simulink model "sys_model"  (R2015a)
settings: configuration reference "config_cosim" (kept outside this file)
InitFcn:
  | h  = findall(0, 'tag','Display');
  | close(h)
  | load TestVel
StartFcn:
  | Display
StopFcn:
  | h  = findall(0, 'tag','Display');
  | %close(h)
undefined symbols (not defined in the file): Vmsl, Vtgt
(part 2 of 2)

== stateflow chart sys_model/CC_module/Subsystem/DisplayControl ==
  settings: executeAtInitialization=1
  state Init
    entry:
    TargetData= TargetDataLD;
    AsnData = zeros(8,2)
    StateData = zeros(8,3);
    StateInf = 0;
    avl_asn_msl = ones(8,1);
    avl_FS_tgt = ones(8,1);
    avl_pwr_tgt = ones(8,1);
  state On
    state TargetPower [parallel]
      % 根据选择的目标更新加电和断电信息
      settings: executionOrder=4
      TargetPower -> (junction 337)
      (junction 337) -> (junction 441) [order 1] : [Actions.TgtAsn]
      (junction 337) -> (junction 339) [order 2]
      (junction 441) -> (junction 443) : {avl_pwr_tgt(Inds.TgtAsnInd) = 1;}
      (junction 443) -> (junction 339)
      (junction 339) -> (junction 687)
      (junction 687) -> (junction 685) [order 1] : [Actions.TgtAsnCcl]
      (junction 687) -> (junction 684) [order 2]
      (junction 685) -> (junction 691) : {avl_pwr_tgt(Inds.TgtAsnInd) = 0;}
      (junction 691) -> (junction 684)
    state DataProcess [parallel]
      en:
      %info2FSC.Para_FS(1:8) = 0;
      Para_FS0.pos_tgt = [0;0;0];
      Para_FS0.vel_tgt = [0;0;0];
      info2FSC.Para_FS(1:8) = Para_FS0;
      info2FSC.ins_pwr_on =  false(8,1);
      info2FSC.ins_pwr_of = [false;false;false;false;false;false;false;false];
      info2FSC.ins_FS = [false;false;false;false;false;false;false;false];
      settings: executionOrder=6
      state PwrOff [parallel]
        settings: executionOrder=3
        (default) -> (junction 889)
        On.DataProcess.PwrOff -> (junction 889)
        (junction 889) -> (junction 880) [order 1] : [Actions.PwrOff]
        (junction 889) -> (junction 1219) [order 2]
        (junction 880) -> (junction 1217) : {info2FSC.ins_pwr_on = [false;false;false;false;false;false;false;false];
            | info2FSC.ins_pwr_of =Inds.PwrInd;
            | info2FSC.ins_FS = [false;false;false;false;false;false;false;false];}
        (junction 1217) -> (junction 1219)
        (junction 1219) -> (junction 1382)
      state PwrOn [parallel]
        settings: executionOrder=1
        (default) -> (junction 863)
        (junction 863) -> (junction 852) [order 1] : [Actions.PwrOn]
        On.DataProcess.PwrOn -> (junction 863)
        (junction 863) -> (junction 1212) [order 2]
        (junction 852) -> (junction 1214) : {info2FSC.ins_pwr_on = Inds.PwrInd;
            | info2FSC.ins_pwr_of = [false;false;false;false;false;false;false;false];
            | info2FSC.ins_FS = [false;false;false;false;false;false;false;false];}
        (junction 1214) -> (junction 1212)
        (junction 1212) -> (junction 1380)
      state FS [parallel]
        settings: executionOrder=2
        (default) -> (junction 914)
        On.DataProcess.FS -> (junction 914)
        (junction 914) -> (junction 905) [order 1] : [Actions.FS]
        (junction 914) -> (junction 1222) [order 2]
        (junction 905) -> (junction 902) : {info2FSC.ins_pwr_on = [false;false;false;false;false;false;false;false];
            | info2FSC.ins_pwr_of = [false;false;false;false;false;false;false;false];
            | info2FSC.ins_FS = [false;false;false;false;false;false;false;false];}
        (junction 913) -> (junction 922) [order 1] : [Inds.TgtFsInd(i,1)]
        (junction 1221) -> (junction 913) [order 1] : [i  < 9]
        (junction 902) -> (junction 1221) : {i = 1;}
        (junction 913) -> (junction 907) [order 2]
        (junction 922) -> (junction 1201) : {ddInd1 = AsnData(i,1);
            | info2FSC.ins_FS(ddInd1) = true;}
        (junction 1201) -> (junction 907)
        (junction 907) -> (junction 919)
        (junction 1221) -> (junction 1222) [order 2]
        (junction 916) -> (junction 1221) : {i = i + 1;}
        (junction 1222) -> (junction 1384)
        (junction 919) -> (junction 918) [order 1] : [Inds.TgtFsInd(i,2)]
        (junction 918) -> (junction 1203) : {ddInd1 = AsnData(i,2);
            | info2FSC.ins_FS(ddInd1) = true;}
        (junction 919) -> (junction 916) [order 2]
        (junction 1203) -> (junction 916)
      state DataUpdateWithFSCInfo [parallel]
        settings: executionOrder=4
        state Enter
        state Sub
          (default) -> (junction 981)
          (junction 981) -> (junction 980) : {avl_asn_msl =double(avl_asn_msl&info_FSC.avl_msl);
              | m = 0;
              | n = 0;
              | j = 1;}
          (junction 979) -> (junction 968) [order 1] : % 导弹出现故障
              | [~info_FSC.avl_msl(j)]
          (junction 980) -> (junction 979) [order 1] : [j  < 9]
          (junction 979) -> (junction 972) [order 2]
          (junction 968) -> (junction 994) : {StateData(j,1:3) =2;}
          (junction 972) -> (junction 984) [order 1] : %虽然有加电命令，但是加电状态为未加电
              | [info2FSC.ins_pwr_on(j)==1 && info_FSC.stt_pwr_msl(j) ==0]
          (junction 977) -> (junction 980) : {j = j + 1;}
          (junction 980) -> (junction 999) [order 2]
          (junction 972) -> (junction 973) [order 2]
          (junction 984) -> (junction 988) : {StateData(j,2) = 0;
              | m = m+1;}
          (junction 973) -> (junction 966) [order 1] : %虽然有发射命令，但是离架计时为0，说明没有发生
              | [info2FSC.ins_FS(j)==1 && info_FSC.count_sprt_msl(j)<=0]
          (junction 973) -> (junction 977) [order 2]
          (junction 966) -> (junction 991) : {StateData(j,3) = 0;
              | n = n+1;}
          (junction 991) -> (junction 977)
          (junction 988) -> (junction 991)
          (junction 994) -> (junction 988)
          (junction 999) -> (junction 1001) [order 1] : [sum(info2FSC.ins_pwr_on)>0&&StateInf~= 712]
          (junction 1001) -> (junction 1350) [order 1] : % 说明本次没有加电成功的DD
              | [m == sum(info2FSC.ins_pwr_on)]
          (junction 999) -> (junction 1005) [order 2]
          (junction 1001) -> (junction 1003) [order 2] : {StateInf = 710;}
          (junction 1350) -> (junction 1352) : {StateInf = 712;}
          (junction 1003) -> (junction 1005)
          (junction 1352) -> (junction 1003)
          (junction 1005) -> (junction 1368)
          (junction 1368) -> (junction 1369) [order 1] : [sum(info2FSC.ins_pwr_of)>0]
          (junction 1368) -> (junction 1370) [order 2]
          (junction 1369) -> (junction 1371) : {StateInf = 810;}
          (junction 1371) -> (junction 1370)
          (junction 1370) -> (junction 1009)
          (junction 1009) -> (junction 1491) [order 1] : [sum(info2FSC.ins_FS)>0]
          (junction 1491) -> (junction 1011) [order 1] : [n == sum(info2FSC.ins_FS)] % 说明本次没有发射成功的DD
          (junction 1009) -> (junction 1008) [order 2]
          (junction 1491) -> (junction 1493) [order 2] : {StateInf = 112;}
          (junction 1011) -> (junction 1012) : {StateInf = 110;}
          (junction 1493) -> (junction 1008)
          (junction 1012) -> (junction 1493)
          (junction 1008) -> (junction 1021) : {StateData0.StateData = StateData;
              | StateData0.StateInf = StateInf;
              | avl_FS_tgt = avl_FS_tgt0;}
        state Waiting
          en:StateInf = 0;
        (default) -> On.DataProcess.DataUpdateWithFSCInfo.Enter
        On.DataProcess.DataUpdateWithFSCInfo.Enter -> On.DataProcess.DataUpdateWithFSCInfo.Waiting : [Actions.PwrOn||Actions.PwrOff||Actions.FS]
        On.DataProcess.DataUpdateWithFSCInfo.Waiting -> Sub : [after(1,tick)]
        Sub -> DataUpdateWithFSCInfo
    state TargetDataProcess [parallel]
      settings: executionOrder=1
      state Time
      (default) -> Time : { TargetData = TargetDataLD;}
      Time -> TargetDataProcess : [after(0.001,sec)]
    state DataUpdate [parallel]
      % 根据状态更新状态信息以及表格中要显示的数据
      en:StateData = zeros(8,3);
      settings: executionOrder=2
      state Assign [parallel]
        settings: executionOrder=1
        Assign -> (junction 412)
        (junction 412) -> (junction 416) [order 1] : [Actions.TgtAsn]
        (junction 412) -> (junction 415) [order 2]
        (junction 416) -> (junction 410) : {AsnData(Inds.TgtAsnInd,1) = Inds.MslInd(1);
            |  AsnData(Inds.TgtAsnInd,2) = Inds.MslInd(2);}
        (junction 410) -> (junction 447) [order 1] : [Inds.MslInd(1)]
        (junction 410) -> (junction 815) [order 2]
        (junction 447) -> (junction 814) : {StateData(Inds.MslInd(1),2)= 1;}
        (junction 814) -> (junction 815)
        (junction 815) -> (junction 449)
        (junction 449) -> (junction 452) [order 1] : [Inds.MslInd(2)]
        (junction 449) -> (junction 454) [order 2]
        (junction 452) -> (junction 818) : {StateData(Inds.MslInd(2),2) = 1;}
        (junction 454) -> (junction 415)
        (junction 818) -> (junction 454)
        (junction 415) -> (junction 662)
        (junction 662) -> (junction 664) [order 1] : [Actions.TgtAsnCcl]
        (junction 662) -> (junction 665) [order 2]
        (junction 664) -> (junction 1518) : {AsnData(Inds.TgtAsnInd,1) = 0;
            |  AsnData(Inds.TgtAsnInd,2) = 0;}
        (junction 1518) -> (junction 1512) [order 1] : [Inds.MslInd(1)]
        (junction 1518) -> (junction 1510) [order 2]
        (junction 1512) -> (junction 1520) : {StateData(Inds.MslInd(1),2) = 0;}
        (junction 1520) -> (junction 1510)
        (junction 1510) -> (junction 1504)
        (junction 1504) -> (junction 1503) [order 1] : [Inds.MslInd(2)]
        (junction 1504) -> (junction 1517) [order 2]
        (junction 1503) -> (junction 1516) : {StateData(Inds.MslInd(2),2) = 0;}
        (junction 1517) -> (junction 665)
        (junction 1516) -> (junction 1517)
        (junction 665) -> (junction 1360) : {StateData0.StateData = StateData;
            | StateData0.StateInf = 0;}
      state PwrOn [parallel]
        settings: executionOrder=2
        state PowerOn
          (default) -> (junction 532) : {i = 1;}
          (junction 544) -> (junction 543) [order 1] : [PwrInd(i)]
          (junction 532) -> (junction 544) [order 1] : [i  < 9]
          (junction 544) -> (junction 545) [order 2]
          (junction 543) -> (junction 542) : {StateData(i,1) = 1;}
          (junction 545) -> (junction 532) : {i = i + 1;}
          (junction 542) -> (junction 545)
          (junction 532) -> (junction 1229) [order 2]
        state Enter
        state Waiting
          entry:
          PwrInd = Inds.PwrInd;
        (default) -> On.DataUpdate.PwrOn.Enter
        On.DataUpdate.PwrOn.Enter -> On.DataUpdate.PwrOn.Waiting : [Actions.PwrOn]
        On.DataUpdate.PwrOn.Waiting -> PowerOn : [after(1,tick)]
        PowerOn -> On.DataUpdate.PwrOn
      state FS [parallel]
        settings: executionOrder=4
        state Enter3
        state Waiting3
          entry:
          TgtFsInd = Inds.TgtFsInd;
        state fs
          (junction 611) -> (junction 604) [order 1] : [i  < 9]
          (junction 604) -> (junction 607)
          (default) -> (junction 611) : {i = 1;}
          (junction 607) -> (junction 608) [order 1] : [TgtFsInd(i,1)>0]
          (junction 607) -> (junction 609) [order 2]
          (junction 608) -> (junction 610) : {ddInd = AsnData(i,1);
              | StateData(ddInd,3) = 1;}
          (junction 610) -> (junction 609)
          (junction 609) -> (junction 612)
          (junction 617) -> (junction 611) : {i = i + 1;}
          (junction 611) -> (junction 616) [order 2]
          (junction 612) -> (junction 613) [order 1] : [TgtFsInd(i,2)>0]
          (junction 612) -> (junction 614) [order 2]
          (junction 613) -> (junction 615) : {ddInd = AsnData(i,2);
              | StateData(ddInd,3) = 1;}
          (junction 615) -> (junction 614)
          (junction 614) -> (junction 617)
        (default) -> Enter3
        Enter3 -> Waiting3 : [Actions.FS]
        Waiting3 -> fs : [after(1,tick)]
        fs -> On.DataUpdate.FS
      state PwrOff [parallel]
        settings: executionOrder=3
        state Enter1
        state Poweroff
          (default) -> (junction 735) : {i = 1;}
          (junction 728) -> (junction 727) [order 1] : [PwrInd(i)]
          (junction 735) -> (junction 728) [order 1] : [i  < 9]
          (junction 728) -> (junction 719) [order 2]
          (junction 727) -> (junction 725) : {StateData(i,1) = 0;}
          (junction 719) -> (junction 735) : {i = i + 1;}
          (junction 725) -> (junction 719)
          (junction 735) -> (junction 1464) [order 2] : {i = 1;}
        state Waiting1
          entry:
          PwrInd = Inds.PwrInd;
        (default) -> Enter1
        Enter1 -> Waiting1 : [Actions.PwrOff]
        Waiting1 -> Poweroff : [after(1,tick)]
        Poweroff -> On.DataUpdate.PwrOff
    state TargetAssign [parallel]
      % 根据选择的目标、FSC和DD更新可分配的目标、FSC和DD数据
      en:avl_asn_tgt = ones(8,1);
      settings: executionOrder=3
      (junction 328) -> (junction 330) [order 1] : [Actions.TgtAsn]
      TargetAssign -> (junction 328)
      (junction 330) -> (junction 421) : {avl_asn_tgt(Inds.TgtAsnInd) = 0;}
      (junction 328) -> (junction 329) [order 2]
      (junction 421) -> (junction 423) [order 1] : [Inds.MslInd(1)>0]
      (junction 421) -> (junction 824) [order 2]
      (junction 423) -> (junction 826) : {avl_asn_msl(Inds.MslInd(1)) = 0;}
      (junction 826) -> (junction 824)
      (junction 824) -> (junction 430)
      (junction 430) -> (junction 436) [order 1] : [Inds.MslInd(2)>0]
      (junction 430) -> (junction 434) [order 2]
      (junction 436) -> (junction 822) : {avl_asn_msl(Inds.MslInd(2)) = 0;}
      (junction 434) -> (junction 329)
      (junction 822) -> (junction 434)
      (junction 329) -> (junction 637)
      (junction 637) -> (junction 655) [order 1] : [Actions.TgtAsnCcl]
      (junction 655) -> (junction 641) : {avl_asn_tgt(Inds.TgtAsnInd) = 1;}
      (junction 637) -> (junction 639) [order 2]
      (junction 641) -> (junction 647) [order 1] : [Inds.MslInd(1)>0]
      (junction 641) -> (junction 831) [order 2]
      (junction 647) -> (junction 830) : {avl_asn_msl(Inds.MslInd(1)) = 1;}
      (junction 830) -> (junction 831)
      (junction 831) -> (junction 646)
      (junction 646) -> (junction 648) [order 1] : [Inds.MslInd(2)>0]
      (junction 648) -> (junction 828) : {avl_asn_msl(Inds.MslInd(2)) = 1;}
      (junction 646) -> (junction 643) [order 2]
      (junction 643) -> (junction 639)
      (junction 828) -> (junction 643)
    state FS [parallel]
      % 根据选择的目标更新DD发射信息,因为断电的时候判断发射可用，
      %需要用到状态表中的数据，有一定延迟，所以放在断电时放在DataUpdate中
      entry:avl_FS_tgt = zeros(8,1);
      avl_FS_tgt0 = zeros(8,1);
      settings: executionOrder=5
      On.FS -> (junction 587)
      (junction 587) -> (junction 585) [order 1] : [Actions.PwrOn]
      (junction 587) -> (junction 693) [order 2]
      (junction 585) -> (junction 577) : {i = 1;}
      (junction 577) -> (junction 590) [order 1] : [i  < 9]
      (junction 577) -> (junction 693) [order 2]
      (junction 590) -> (junction 597) [order 1] : [Inds.PwrInd(i)]
      (junction 571) -> (junction 577) : {i = i + 1;}
      (junction 693) -> (junction 707)
      (junction 590) -> (junction 571) [order 2]
      (junction 597) -> (junction 1185) : {avl_FS_tgt0(i) = 1;}
      (junction 1185) -> (junction 571)
  (default) -> Init
  Init -> On : after(0.001,sec)
  data: pos function_input double size=[8 3]; l function_output double size=8; TargetDataLD input Bus: TgtDataLDBusObject size=1; TargetData output Bus: TgtDataLDBusObject size=1; AsnData output size=[8 2]; avl_asn_tgt output double size=8; avl_asn_msl output double size=8; avl_pwr_tgt output double size=8; avl_FS_tgt output double size=8; StateData0 output Bus: StateBusObject; i local; ddInd local; info2FSC output Bus: BusObject_info_CC2FSC size=1; ddInd1 local; Actions input Bus: ActionBusObject size=1; info_FSC input Bus: BusObject_info_FSC2CC size=1; StateData local double size=[8 3]; StateInf local double size=1; m local; n local; j local; DD1 local; DD2 local; Para_FS0 local Bus: BusObject_msg_FSC2msl; DD10 local; DD20 local; avl_FS_tgt0 local; L local double size=8; Inds input Bus: ChooseBusObject; TgtFsInd local double size=[8 2]; PwrInd local boolean
  function l = PosCal(pos):
    | function l = PosCal(pos)
    | l = zeros(8,1);
    | for i = 1:8
    | l(i) =sqrt( pos(i,1)^2 + pos(i,2)^2);
    | end

== stateflow chart sys_model/CC_module/Subsystem/Subsystem/Chart1 ==
  state maintain
    % 保持已有速度，更新新的导弹速度
    (default) -> (junction 53)
    maintain -> (junction 53)
    (junction 53) -> (junction 8) : %导弹循环
        | {i = 1;}
    (junction 8) -> (junction 15) [order 1] : [i<8]
    (junction 15) -> (junction 37) [order 1] : [FSMsltgtInd(i)]
    (junction 14) -> (junction 8) : {i = i+1;}
    (junction 8) -> (junction 51) [order 2]
    (junction 15) -> (junction 14) [order 2]
    (junction 37) -> (junction 19) : { aa = MslMotionNew.Pos(i,:);
        | MslMotion.Pos(i,:) =MslMotionNew.Pos(i,:);
        | MslMotion.Vel(i,:) = MslMotionNew.Vel(i,:);}
    (junction 19) -> (junction 14)
  (default) -> maintain : % 由导弹发射信息、其对应的目标和导弹的运动更新导弹的运动
      |
      | {MslMotion.Pos =  zeros(8,2);
      | MslMotion.Vel =  zeros(8,2);}
  data: FSMsltgtInd input double size=8; MslMotionNew input Bus: MslDataBusObject size=1; MslMotion output Bus: MslDataBusObject size=1; i local; aa local

== stateflow chart sys_model/CC_module/Subsystem/Subsystem/Chart ==
  (default) -> (junction 9) : % 由分配的目标得到导弹对应的目标
      |
      | {MsltgtInd = zeros(8,1);
      | FSMsltgtInd = zeros(8,1);}
  (junction 9) -> (junction 10) : %导弹循环
      | {i = 1;}
  (junction 21) -> (junction 38) [order 1] : [AsnData(j,1) == i]
  (junction 31) -> (junction 21) [order 1] : [j<8]
  (junction 21) -> (junction 42) [order 2]
  (junction 38) -> (junction 44) : {MsltgtInd(i) = j;}
  (junction 10) -> (junction 23) [order 1] : [i<8]
  (junction 11) -> (junction 10) : {i = i+1;}
  (junction 10) -> (junction 59) [order 2]
  (junction 23) -> (junction 31) : %目标循环
      | {j = 1;}
  (junction 50) -> (junction 31) : {j = j+1;}
  (junction 31) -> (junction 70) [order 2]
  (junction 44) -> (junction 42)
  (junction 42) -> (junction 46)
  (junction 46) -> (junction 51) [order 1] : [AsnData(j,2) == i]
  (junction 46) -> (junction 50) [order 2]
  (junction 51) -> (junction 49) : {MsltgtInd(i) = j;}
  (junction 70) -> (junction 71) [order 1] : [ins_fs(i) ]
  (junction 70) -> (junction 11) [order 2]
  (junction 71) -> (junction 73) : {FSMsltgtInd(i) = MsltgtInd(i);}
  (junction 49) -> (junction 50)
  (junction 73) -> (junction 11)
  data: AsnData input size=[8 2]; MsltgtInd output double size=8; FSMsltgtInd output; ins_fs input size=8; i local; j local
